simulink model "MultiportSwitch_TestGen16"  (R2017b)
settings: Solver=FixedStepDiscrete  StartTime=0.0  StopTime=10.0  RelTol=1e-3
undefined symbols (not defined in the file): Block_TestLib, enable_trigger
settings Model: Creator=ktrinh  LastModifiedBy=ktrinh
settings DebuggingCC: ParameterOverflowMsg=none

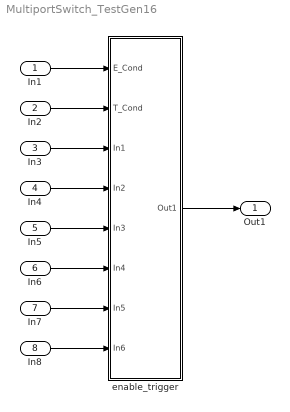
== system MultiportSwitch_TestGen16 ==
  In1 : Inport
  In2 : Inport  Port=2
  In3 : Inport  Port=3
  In4 : Inport  Port=4
  In5 : Inport  Port=5
  In6 : Inport  Port=6
  In7 : Inport  Port=7
  In8 : Inport  Port=8
  enable_trigger : Subsystem  AncestorBlock=Block_TestLib/enable_trigger
  Out1 : Outport
  wires:
  In1/1 -> enable_trigger/1(E_Cond)
  In2/1 -> enable_trigger/2(T_Cond)
  In3/1 -> enable_trigger/3(In1)
  In4/1 -> enable_trigger/4(In2)
  In5/1 -> enable_trigger/5(In3)
  In6/1 -> enable_trigger/6(In4)
  In7/1 -> enable_trigger/7(In5)
  In8/1 -> enable_trigger/8(In6)
  enable_trigger/1(Out1) -> Out1/1

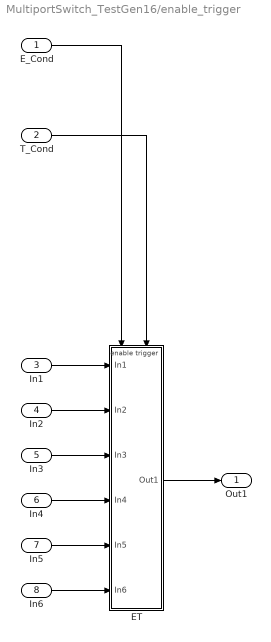
== system MultiportSwitch_TestGen16/enable_trigger ==
  E_Cond : Inport  OutDataTypeStr=boolean
  T_Cond : Inport  Port=2  OutDataTypeStr=boolean
  In1 : Inport  Port=3
  In2 : Inport  Port=4
  In3 : Inport  Port=5
  In4 : Inport  Port=6
  In5 : Inport  Port=7
  In6 : Inport  Port=8
  ET : Subsystem  TreatAsAtomicUnit=on
  Out1 : Outport
  wires:
  T_Cond/1 -> ET/Trigger
  E_Cond/1 -> ET/Enable
  In1/1 -> ET/1(In1)
  In2/1 -> ET/2(In2)
  In3/1 -> ET/3(In3)
  In4/1 -> ET/4(In4)
  In5/1 -> ET/5(In5)
  In6/1 -> ET/6(In6)
  ET/1(Out1) -> Out1/1

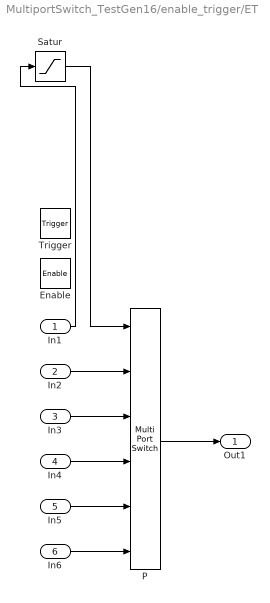
== system MultiportSwitch_TestGen16/enable_trigger/ET ==
  In1 : Inport  OutMin=1  OutMax=5
  In2 : Inport  Port=2  PortDimensions=[2,3]
  In3 : Inport  Port=3  PortDimensions=[2,3]
  In4 : Inport  Port=4  PortDimensions=[2,3]
  In5 : Inport  Port=5  PortDimensions=[2,3]
  In6 : Inport  Port=6  PortDimensions=[2,3]
  Enable : EnablePort
  Trigger : TriggerPort  VariantControl=Variant
  P : MultiPortSwitch  Inputs=4  DataPortForDefault=Additional data port
  Satur : Saturate  UpperLimit=5  LowerLimit=1
  Out1 : Outport
  wires:
  In2/1 -> P/2
  In3/1 -> P/3
  In4/1 -> P/4
  In5/1 -> P/5
  In6/1 -> P/6
  P/1 -> Out1/1
  In1/1 -> Satur/1
  Satur/1 -> P/1
